simulink model "rtwdemo_tflfixpt"  (Simulink 7.6)
settings: Solver=ode3  StartTime=0.0  StopTime=20  FixedStep=.01  RelTol=1e-3  SampleTimeConstraint=Specified
PreLoadFcn:
  | addpath(fullfile(matlabroot,'toolbox','rtw','rtwdemos','tfl_demo'));
  | sl_refresh_customizations;
libraries: rtwdemowidgets x2
settings Model: Creator=The MathWorks Inc.  ExtModeAutoUpdateStatusClock=off
settings MATStruct: SampleTime=1  Offset=0  Priority=[30.0]
settings DataIOCC: SaveOutput=off  SaveTime=off  SignalLoggingName=sigsOut
settings OptimizationCC: InlineParams=on  InlineInvariantSignals=on  PassReuseOutputArgsAs=Individual arguments  StateBitsets=on  DataBitsets=on  UseTempVars=on  ZeroExternalMemoryAtStartup=off  ZeroInternalMemoryAtStartup=off  NoFixptDivByZeroProtection=on  EfficientFloat2IntCast=on  EfficientMapNaN2IntZero=off  OptimizeModelRefInitCode=on  LifeSpan=1
settings DebuggingCC: CheckExecutionContextPreStartOutputMsg=on  CheckExecutionContextRuntimeOutputMsg=on  SolverPrmCheckMsg=none  IntegerOverflowMsg=none  ParameterPrecisionLossMsg=none  StrictBusMsg=ErrorOnBusTreatedAsVector
settings HardwareCC: ProdIntDivRoundTo=Zero  ProdEndianess=LittleEndian  ProdHWDeviceType=Generic->32-bit Embedded Processor  TargetHWDeviceType=32-bit Generic
settings SFSimCC: SFSimEnableDebug=off  SFSimOverflowDetection=off  SimParseCustomCode=off
settings RTWCC: SystemTargetFile=ert.tlc  GenCodeOnly=on  TemplateMakefile=ert_default_tmf  Description=Real-Time Workshop Embedded Coder (no auto configuration)  GenerateReport=on  RTWVerbose=off  ProcessScript=ert_make_rtw_hook  IncludeHyperlinkInReport=on  LaunchReport=on
settings CodeAppCC: ForceParamTrailComments=on  IgnoreCustomStorageClasses=off  IgnoreTestpoints=on  SimulinkDataObjDesc=on  CustomSymbolStrGlobalVar=rt$N$M  CustomSymbolStrType=$N$M  CustomSymbolStrFcn=$N$M$F  CustomSymbolStrMacro=$N$M  InsertBlockDesc=on
settings ERTTargetCC: TargetFunctionLibrary=Fixed Point Examples  MultiwordLength=2048  GenerateSampleERTMain=on  IncludeMdlTerminateFcn=off  SupportNonFinite=off  SupportComplex=off  InlinedParameterPlacement=NonHierarchical  ERTCustomFileTemplate=example_file_process.tlc  ConvertIfToSwitch=off

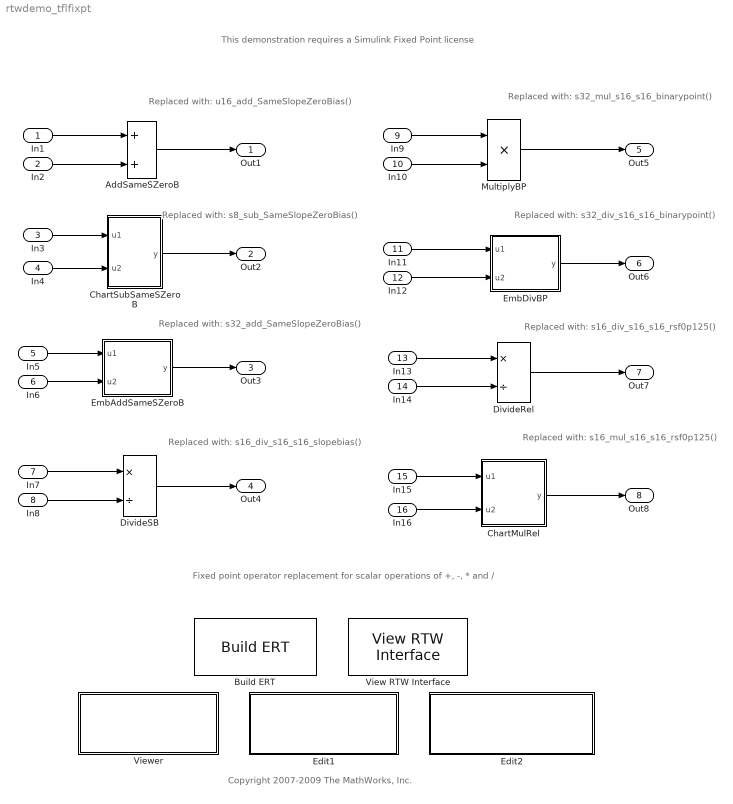
== system rtwdemo_tflfixpt ==
  note: This demonstration requires a Simulink Fixed Point license
  note: Copyright 2007-2009 The MathWorks, Inc.
  note: Fixed point operator replacement for scalar operations of +, -, * and /
  note: Replaced with:
      | u16_add_SameSlopeZeroBias()
  note: Replaced with:
      | s16_div_s16_s16_rsf0p125()
  note: Replaced with:
      | s32_div_s16_s16_binarypoint()
  note: Replaced with:
      | s16_div_s16_s16_slopebias()
  note: Replaced with:
      | s16_mul_s16_s16_rsf0p125()
  note: Replaced with:
      | s32_mul_s16_s16_binarypoint()
  note: Replaced with:
      | s32_add_SameSlopeZeroBias()
  note: Replaced with:
      | s8_sub_SameSlopeZeroBias()
  In1 : Inport  OutDataTypeStr=fixdt(0,16,13)  PortDimensions=1  SampleTime=1  Interpolate=off
  In2 : Inport  Port=2  OutDataTypeStr=fixdt(0,16,13)  PortDimensions=1  SampleTime=1  Interpolate=off
  In3 : Inport  Port=3  OutDataTypeStr=fixdt(1,8,5)  PortDimensions=1  SampleTime=1  Interpolate=off
  In4 : Inport  Port=4  OutDataTypeStr=fixdt(1,8,5)  PortDimensions=1  SampleTime=1  Interpolate=off
  In5 : Inport  Port=5  OutDataTypeStr=fixdt(1,32,2^-15,0)  PortDimensions=1  SampleTime=1
  In6 : Inport  Port=6  OutDataTypeStr=fixdt(1,32,2^-15,0)  PortDimensions=1  SampleTime=1
  In7 : Inport  Port=7  OutDataTypeStr=fixdt(1,16,15,2)  PortDimensions=1  SampleTime=1  Interpolate=off
  In8 : Inport  Port=8  OutDataTypeStr=fixdt(1,16,13,5)  PortDimensions=1  SampleTime=1  Interpolate=off
  In9 : Inport  Port=9  OutDataTypeStr=fixdt(1,16,15)  PortDimensions=1  SampleTime=1  Interpolate=off
  In10 : Inport  Port=10  OutDataTypeStr=fixdt(1,16,13)  PortDimensions=1  SampleTime=1  Interpolate=off
  In11 : Inport  Port=11  OutDataTypeStr=fixdt(1,16,15)  PortDimensions=1  SampleTime=1  Interpolate=off
  In12 : Inport  Port=12  OutDataTypeStr=fixdt(1,16,13)  PortDimensions=1  SampleTime=1  Interpolate=off
  In13 : Inport  Port=13  OutDataTypeStr=int16  PortDimensions=1  SampleTime=1  Interpolate=off
  In14 : Inport  Port=14  OutDataTypeStr=fixdt(1,16,-5)  PortDimensions=1  SampleTime=1  Interpolate=off
  In15 : Inport  Port=15  OutDataTypeStr=fixdt(1,16,13)  PortDimensions=1  SampleTime=1
  In16 : Inport  Port=16  OutDataTypeStr=fixdt(1,16,5)  PortDimensions=1  SampleTime=1
  AddSameSZeroB : Sum  RndMeth=Zero
  Build ERT : rtwdemowidgets/Build ERT  SystemSampleTime=-1  attrib_overrides={'GenFloatMathFcnCalls'}
  ChartMulRel : Stateflow chart  TreatAsAtomicUnit=on
  ChartSubSameSZeroB : Stateflow chart  TreatAsAtomicUnit=on
  DivideRel : Product  Inputs=*/  OutDataTypeStr=fixdt(1,16,-13)  RndMeth=Ceiling
  DivideSB : Product  Inputs=*/  OutDataTypeStr=Inherit: Inherit via back propagation  RndMeth=Ceiling  SaturateOnIntegerOverflow=on
  Edit1 : Subsystem  mask{attrib_overrides={}}
      mask prompts: attrib_overrides "List of attributes to preserve (cell of strings):"
      mask help: Enter the attributes of the configuration set that you want preserved. Otherwise, the default configuration script will override your current settings.
      settings: OpenFcn=edit('tfl_table_fixpt');
      mask Display:
      | disp(['View/edit TFL Definition\n',...
      | 	  'tfl_table_fixpt.m\n(double-click)'])
  Edit2 : Subsystem  mask{attrib_overrides={}}
      mask prompts: attrib_overrides "List of attributes to preserve (cell of strings):"
      mask help: Enter the attributes of the configuration set that you want preserved. Otherwise, the default configuration script will override your current settings.
      settings: OpenFcn=edit(fullfile(matlabroot,'toolbox','rtw','rtwdemos','tfl_demo', 'sl_customization.m'));
      mask Display:
      | disp(['View/edit TFL Registration\n',...
      | 	  'sl_customization.m\n(double-click)'])
  EmbAddSameSZeroB : Stateflow chart  TreatAsAtomicUnit=on
  EmbDivBP : Stateflow chart  TreatAsAtomicUnit=on
  MultiplyBP : Product  OutDataTypeStr=fixdt(1,32,28)  SaturateOnIntegerOverflow=on  RndMeth=Zero
  View RTW Interface : rtwdemowidgets/View RTW Interface  SystemSampleTime=-1
  Viewer : Subsystem  mask{attrib_overrides={}}
      mask prompts: attrib_overrides "List of attributes to preserve (cell of strings):"
      mask help: Enter the attributes of the configuration set that you want preserved. Otherwise, the default configuration script will override your current settings.
      settings: OpenFcn=|
      | tfl = tfl_table_fixpt;
      | obj = RTW.viewTfl(tfl);
      | clear tfl obj;
      mask Display:
      | disp(['Invoke TFL Viewer on\n',...
      | 	  'tfl_table_fixpt.m\n(double-click)'])
  Out1 : Outport
  Out2 : Outport  Port=2
  Out3 : Outport  Port=3  OutDataTypeStr=fixdt(1,32,2^-15,0)
  Out4 : Outport  Port=4
  Out5 : Outport  Port=5
  Out6 : Outport  Port=6
  Out7 : Outport  Port=7
  Out8 : Outport  Port=8
  wires:
  AddSameSZeroB/1 -> Out1/1
  In1/1 -> AddSameSZeroB/1
  In2/1 -> AddSameSZeroB/2
  ChartSubSameSZeroB/1(y) -> Out2/1
  In5/1 -> EmbAddSameSZeroB/1(u1)
  In6/1 -> EmbAddSameSZeroB/2(u2)
  EmbAddSameSZeroB/1(y) -> Out3/1
  In13/1 -> DivideRel/1
  In14/1 -> DivideRel/2
  In9/1 -> MultiplyBP/1
  In10/1 -> MultiplyBP/2
  DivideRel/1 -> Out7/1
  MultiplyBP/1 -> Out5/1
  DivideSB/1 -> Out4/1
  In7/1 -> DivideSB/1
  In8/1 -> DivideSB/2
  In15/1 -> ChartMulRel/1(u1)
  In11/1 -> EmbDivBP/1(u1)
  ChartMulRel/1(y) -> Out8/1
  EmbDivBP/1(y) -> Out6/1
  In3/1 -> ChartSubSameSZeroB/1(u1)
  In4/1 -> ChartSubSameSZeroB/2(u2)
  In16/1 -> ChartMulRel/2(u2)
  In12/1 -> EmbDivBP/2(u2)

== system rtwdemo_tflfixpt/Edit1 ==

== system rtwdemo_tflfixpt/Edit2 ==

== system rtwdemo_tflfixpt/Viewer ==

== stateflow chart ChartSubSameSZeroB ==
  (default) -> (junction 3) : {y := u1-u2;}
  data: u1 input fixdt(1,8,5); u2 input fixdt(1,8,5); y output fixdt(1,8,5)

== matlab function EmbAddSameSZeroB ==
  data: u1 input fixdt(1,32,15); y output fixdt(1,32,15); u2 input fixdt(1,32,15)
function y = fcn(u1, u2)
% This block supports the Embedded MATLAB subset.
% See the help menu for details. 

y = u1+u2;

== stateflow chart ChartMulRel ==
  (default) -> (junction 18) : {y := u1*u2;}
  data: u1 input int16; u2 input double =1; y output int16

== matlab function EmbDivBP ==
  settings: fimath=|
      | fimath(...
      | 'RoundMode', 'nearest',...
      | 'OverflowMode', 'saturate',...
      | 'ProductMode', 'KeepLSB', 'ProductWordLength', 32,...
      | 'SumMode', 'KeepLSB', 'SumWordLength', 32,...
      | 'CastBeforeSum', true)
  data: u1 input uint32; y output uint32; u2 input uint32
function y = fcn(u1, u2)
% This block supports the Embedded MATLAB subset.
% See the help menu for details. 

T = numerictype('Signed',true,'Wordlength',32,'Fractionlength',28');
if (u2 == 0)
    y = fi(u1,T);
else
    y = divide(T,u1,u2);
end
